simulink model "ur5_simulink_ros2_pbvs_aic"  (R2023b)
settings: Solver=ode4  StartTime=0.0  StopTime=inf  FixedStep=0.005  RelTol=1e-3
model workspace (MAT data in the model file):
  SL_ROS_VariableLengthArrays_MaxSizes.CommonInfo.ArrayTruncateAction = 'EmitWarning'
  SL_ROS_VariableLengthArrays_MaxSizes.MsgTypeMap = containers.Map
  SL_ROS_VariableLengthArrays_MaxSizes.MsgTypeMap.serialization.keys = {'example_interfaces/Float64MultiArray'}
  SL_ROS_VariableLengthArrays_MaxSizes.MsgTypeMap.serialization.values{1}.PropertyName = 'data'
  SL_ROS_VariableLengthArrays_MaxSizes.MsgTypeMap.serialization.values{1}.DataType = 'double'
  SL_ROS_VariableLengthArrays_MaxSizes.MsgTypeMap.serialization.values{1}.MaxLength = 1
  SL_ROS_VariableLengthArrays_MaxSizes.MsgTypeMap.serialization.uniformity = 0
  SL_ROS_VariableLengthArrays_MaxSizes.MsgTypeMap.serialization.keyType = 'char'
  SL_ROS_VariableLengthArrays_MaxSizes.MsgTypeMap.serialization.valueType = 'any'
values from neighbouring files (symbols this model uses):
  D = zeros(6,12)    [ibvs_cstate.m]
undefined symbols (not defined in the file or in its folder): data, data_SL_Info
libraries: ros2lib x8, simulink x3, robotmaniplib x3, robotcorelib x2
settings Model: SimulationMode=accelerator  Creator=81232  LastModifiedBy=ias-lab-701
settings OptimizationCC: EnhancedBackFolding=on  PassReuseOutputArgsAs=Individual arguments  ZeroExternalMemoryAtStartup=off  ZeroInternalMemoryAtStartup=off  MaxStackSize=64  OptimizeBlockOrder=speed  DifferentSizesBufferReuse=on  OptimizationCustomize=off  EfficientTunableParamExpr=on
settings DebuggingCC: ParameterTunabilityLossMsg=error
settings ModelReferenceCC: EnableRefExpFcnMdlSchedulingChecks=on
settings SFSimCC: MATLABDynamicMemAlloc=off
settings RTWCC: Description=Embedded Coder  SystemTargetFile=ert.tlc  HardwareBoard=Robot Operating System 2 (ROS 2)  TLCOptions="-aInlineSetEventsForThisBaseRateFcn=TLC_FALSE -aSuppressMultiTaskScheduler=TLC_FALSE  -aRateBasedStepFcn=0"  TemplateMakefile=ert_default_tmf  Toolchain=Colcon Tools  TargetLang=C++
settings CodeAppCC: ForceParamTrailComments=on  IgnoreCustomStorageClasses=off  OperatorAnnotations=on  SimulinkDataObjDesc=on  SFDataObjDesc=on  InsertBlockDesc=on
settings ERTTargetCC: CodeInterfacePackaging=C++ class  RootIOFormat=Structure reference

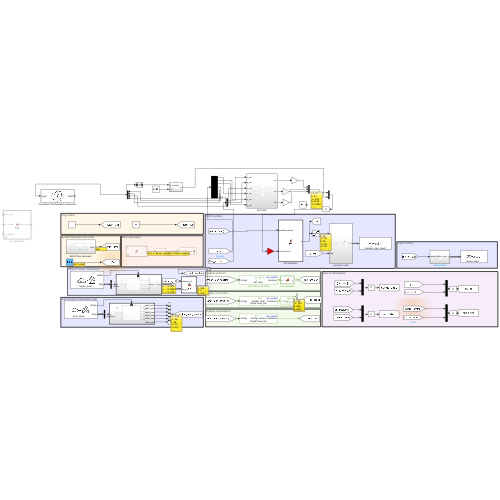
[thumbnail: Simulink's stored preview of the top-level diagram]
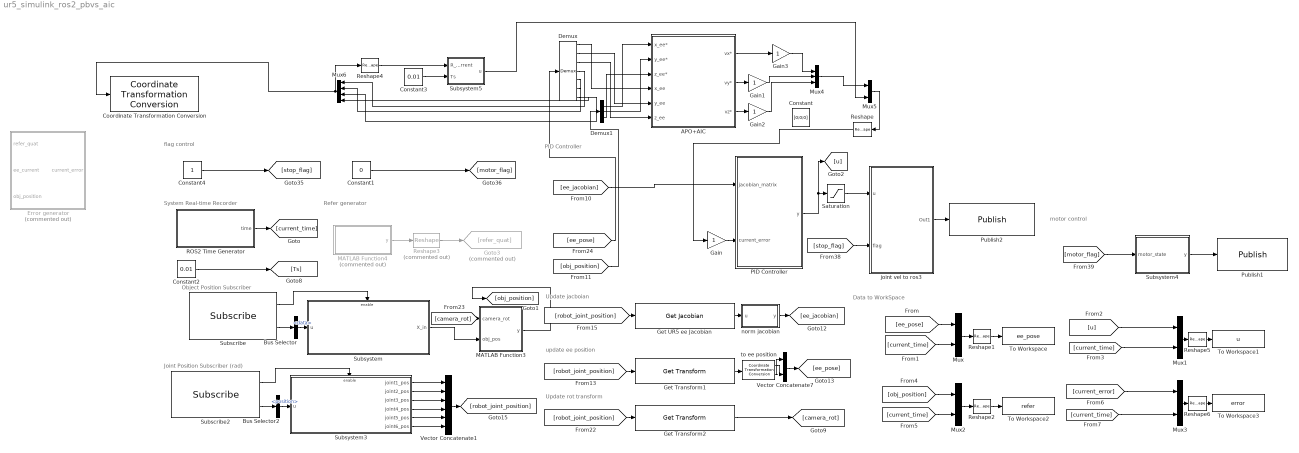
== system ur5_simulink_ros2_pbvs_aic ==
  note: PID Controller
  note: update ee position
  note: Joint Position Subscriber (rad)
  note: Refer generator
  note: Data to WorkSpace
  note: System Real-time Recorder
  note: Object Position Subscriber
  note: Update jacboian
  note: Update rot transform
  note: flag control
  note: motor control
  APO+AIC : Subsystem
  Bus Selector : BusSelector  OutputSignals=data
  Bus Selector2 : BusSelector  OutputSignals=position
  Constant : Constant  Value=[0;0;0]
  Constant1 : Constant  Value=0
  Constant2 : Constant  Value=0.01
  Constant3 : Constant  Value=0.01
  Constant4 : Constant
  Coordinate Transformation Conversion : robotcorelib/Coordinate Transformation Conversion  InputRepresentation=Quaternion  InputEulerSequence=ZYX  ShowTrVecInputPort=on  OutputRepresentation=Rotation Matrix  OutputEulerSequence=ZYX  ShowTrVecOutputPort=on  SimulateUsing=Interpreted execution
  Demux : Demux  Outputs=7
  Demux1 : Demux  Outputs=3
  Error generator : MATLAB Function  Commented=on  TreatAsAtomicUnit=on
  Gain{,1..3} (4 alike) : Gain
  Get Transform1 : robotmaniplib/Get Transform  RigidBodyTree=ur5_model  SourceBody=tool0  TargetBody=base_link  SimulateUsing=Interpreted execution
  Get Transform2 : robotmaniplib/Get Transform  RigidBodyTree=ur5_model  SourceBody=camera  TargetBody=base_link  SimulateUsing=Interpreted execution
  Get UR5 ee Jacobian : robotmaniplib/Get Jacobian  RigidBodyTree=ur5_model  EndEffector=tool0  SimulateUsing=Interpreted execution
  Goto3 : Goto  Commented=on  GotoTag=refer_quat
  MATLAB Function3 : MATLAB Function  TreatAsAtomicUnit=on
  MATLAB Function4 : MATLAB Function  Commented=on  TreatAsAtomicUnit=on
  Mux{,1..3,5} (5 alike) : Mux  Inputs=2
  Mux4 : Mux  Inputs=3
  Mux6 : Mux
  PID Controller : MATLAB Function  TreatAsAtomicUnit=on
  Publish1 : ros2lib/Publish  topicSource=Select from ROS network  topic=/motor_state  messageType=std_msgs/Int64  QOSHistory=Keep last  QOSDepth=1  QOSReliability=Reliable  QOSDurability=Volatile
      settings: LibrarySourceBlock=roslib/ROS 2/Publish
  Publish2 : ros2lib/Publish  topicSource=Select from ROS network  topic=/simulink_mpc_result  messageType=std_msgs/Float64MultiArray  QOSHistory=Keep last  QOSDepth=1  QOSReliability=Reliable  QOSDurability=Volatile
      settings: LibrarySourceBlock=roslib/ROS 2/Publish
  ROS2 Time Generator : Subsystem
  Reshape : Reshape  OutputDimensionality=Customize  OutputDimensions=[6,1]
  Reshape1 : Reshape  OutputDimensionality=Customize  OutputDimensions=[8]
  Reshape2 : Reshape  OutputDimensionality=Customize  OutputDimensions=[4]
  Reshape3 : Reshape  Commented=on  OutputDimensions=[1,7]
  Reshape4 : Reshape  OutputDimensionality=Row vector (2-D)
  Reshape5 : Reshape  OutputDimensionality=Customize  OutputDimensions=[7]
  Reshape6 : Reshape  OutputDimensionality=Customize  OutputDimensions=[7]
  Saturation : Saturate  UpperLimit=0.05  LowerLimit=-0.05  LinearizeAsGain=off
  Subscribe : ros2lib/Subscribe  topicSource=Select from ROS network  topic=/object_pose  messageType=std_msgs/Float64MultiArray  sampleTime=-1  QOSHistory=Keep last  QOSDepth=1  QOSReliability=Reliable  QOSDurability=Volatile
  Subscribe2 : ros2lib/Subscribe  topicSource=Select from ROS network  topic=/joint_states  messageType=sensor_msgs/JointState  sampleTime=-1  QOSHistory=Keep last  QOSDepth=1  QOSReliability=Reliable  QOSDurability=Volatile
  Subsystem : Subsystem
  Subsystem3 : Subsystem
  Subsystem4 : Subsystem
  Subsystem5 : Subsystem
  To Workspace : ToWorkspace  VariableName=ee_pose  SaveFormat=Timeseries  SampleTime=-1
  To Workspace1 : ToWorkspace  VariableName=u  SaveFormat=Timeseries  SampleTime=-1
  To Workspace2 : ToWorkspace  VariableName=refer  SaveFormat=Timeseries  SampleTime=-1
  To Workspace3 : ToWorkspace  VariableName=error  SaveFormat=Timeseries  SampleTime=-1
  Vector Concatenate1 : Concatenate  NumInputs=6
  Vector Concatenate7 : Concatenate
  joint vel to ros3 : Subsystem
  norm jacobian : MATLAB Function  TreatAsAtomicUnit=on
  to ee position : robotcorelib/Coordinate Transformation Conversion  InputRepresentation=Homogeneous Transformation  InputEulerSequence=ZYX  ShowTrVecInputPort=on  OutputRepresentation=Quaternion  OutputEulerSequence=ZYX  ShowTrVecOutputPort=on  SimulateUsing=Interpreted execution
  wires:
  Bus Selector/1 -> Subsystem/1(u)  "<data>"
  Subscribe/2 -> Bus Selector/1
  Subscribe/1 -> Subsystem/Enable
  ROS2 Time Generator/1(time) -> [current_time]
  [ee_pose] -> Mux/1
  [current_time] -> Mux/2
  [current_time] -> Mux1/2
  [current_time] -> Mux2/2
  Mux2/1 -> Reshape2/1
  [current_time] -> Mux3/2
  Mux3/1 -> Reshape6/1
  [current_error] -> Mux3/1
  [u] -> Mux1/1
  Mux1/1 -> Reshape5/1
  Reshape5/1 -> To Workspace1/1
  Reshape6/1 -> To Workspace3/1
  Subscribe2/2 -> Bus Selector2/1
  Bus Selector2/1 -> Subsystem3/1(u)  "<position>"
  Subscribe2/1 -> Subsystem3/Enable
  Subsystem3/1(joint1_pos) -> Vector Concatenate1/1
  Subsystem3/2(joint2_pos) -> Vector Concatenate1/2
  Subsystem3/3(joint3_pos) -> Vector Concatenate1/3
  Subsystem3/4(joint4_pos) -> Vector Concatenate1/4
  Subsystem3/5(joint5_pos) -> Vector Concatenate1/5
  Subsystem3/6(joint6_pos) -> Vector Concatenate1/6
  norm jacobian/1(y) -> [ee_jacobian]
  Get UR5 ee Jacobian/1 -> norm jacobian/1(u)
  [robot_joint_position] -> Get UR5 ee Jacobian/1
  [robot_joint_position] -> Get Transform1/1
  Vector Concatenate1/1 -> [robot_joint_position]
  Mux/1 -> Reshape1/1
  Reshape1/1 -> To Workspace/1
  Reshape2/1 -> To Workspace2/1
  [obj_position] -> Mux2/1
  Constant2/1 -> [Ts]
  Get Transform2/1 -> [camera_rot]
  MATLAB Function3/1(y) -> [obj_position]
  [camera_rot] -> MATLAB Function3/1(camera_rot)
  Subsystem/1(X_in) -> MATLAB Function3/2(obj_pos)
  Reshape3/1 -> Goto3/1
  MATLAB Function4/1(y) -> Reshape3/1
  Get Transform1/1 -> to ee position/1
  to ee position/1 -> Vector Concatenate7/2
  to ee position/2 -> Vector Concatenate7/1
  Vector Concatenate7/1 -> [ee_pose]
  [ee_jacobian] -> PID Controller/1(jacobian_matrix)
  Saturation/1 -> joint vel to ros3/1(u)
  joint vel to ros3/1(Out1) -> Publish2/1
  PID Controller/1(y) -> Saturation/1, [u]
  Constant4/1 -> [stop_flag]
  [stop_flag] -> joint vel to ros3/2(flag)
  Mux5/1 -> Reshape/1
  Gain/1 -> PID Controller/2(current_error)
  Subsystem4/1(y) -> Publish1/1
  [motor_flag] -> Subsystem4/1(motor_state)
  Constant1/1 -> [motor_flag]
  [robot_joint_position] -> Get Transform2/1
  Demux/1 -> APO+AIC/4(x_ee)
  Demux/2 -> APO+AIC/5(y_ee)
  Demux/3 -> APO+AIC/6(z_ee)
  Demux1/1 -> APO+AIC/1(x_ee*)
  Demux1/2 -> APO+AIC/2(y_ee*)
  Demux1/3 -> APO+AIC/3(z_ee*)
  APO+AIC/1(vx*) -> Gain3/1
  APO+AIC/3(vz*) -> Gain2/1
  Mux4/1 -> Mux5/1
  Reshape/1 -> Gain/1
  [ee_pose] -> Demux/1
  [obj_position] -> Demux1/1
  APO+AIC/2(vy*) -> Gain1/1
  Gain1/1 -> Mux4/2
  Gain2/1 -> Mux4/3
  Gain3/1 -> Mux4/1
  Constant3/1 -> Subsystem5/2(Ts)
  Demux/4 -> Mux6/1
  Demux/5 -> Mux6/2
  Demux/6 -> Mux6/3
  Demux/7 -> Mux6/4
  Mux6/1 -> Reshape4/1, Coordinate Transformation Conversion/1
  Subsystem5/1(u) -> Mux5/2
  Reshape4/1 -> Subsystem5/1(R_current)

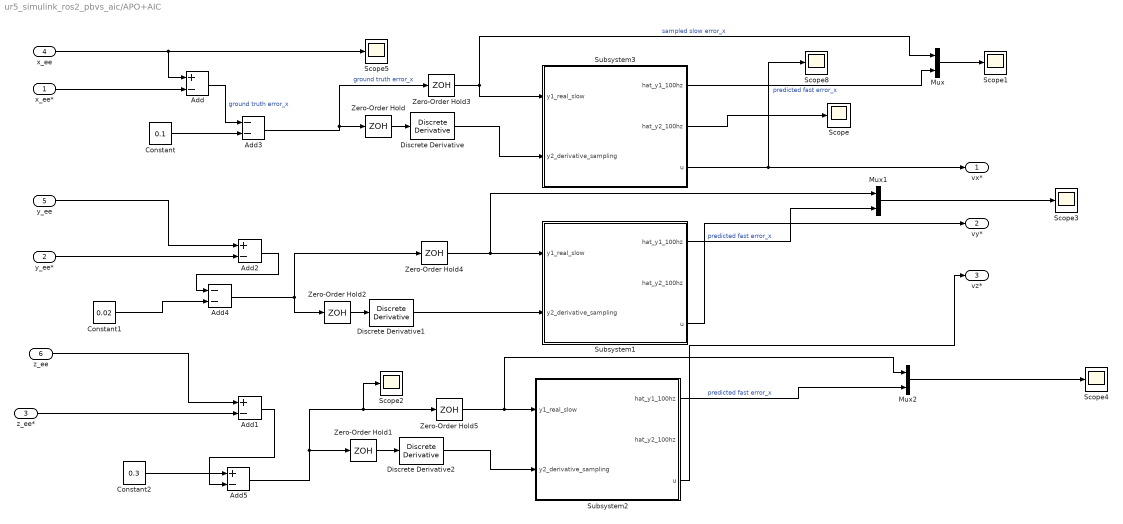
== system ur5_simulink_ros2_pbvs_aic/APO+AIC ==
  x_ee* : Inport
  y_ee* : Inport  Port=2
  z_ee* : Inport  Port=3
  x_ee : Inport  Port=4
  y_ee : Inport  Port=5
  z_ee : Inport  Port=6
  Add{,1..2,5} (4 alike) : Sum  Inputs=+-
  Add3 : Sum  Inputs=--
  Add4 : Sum  Inputs=--
  Constant : Constant  Value=0.1
  Constant1 : Constant  Value=0.02
  Constant2 : Constant  Value=0.3
  Discrete Derivative : simulink/Discrete/Discrete Derivative  gainval=1.0  ICPrevScaledInput=0  OutMin=[]  OutMax=[]  OutDataType=fixdt(1, 16)  OutScaling=2^-10  DoSatur=off
  Discrete Derivative1 : simulink/Discrete/Discrete Derivative  gainval=1.0  ICPrevScaledInput=0.0  OutMin=[]  OutMax=[]  OutDataType=fixdt(1, 16)  OutScaling=2^-10  DoSatur=off
  Discrete Derivative2 : simulink/Discrete/Discrete Derivative  gainval=1.0  ICPrevScaledInput=0.0  OutMin=[]  OutMax=[]  OutDataType=fixdt(1, 16)  OutScaling=2^-10  DoSatur=off
  Mux : Mux  Inputs=2
  Mux1 : Mux  Inputs=2
  Mux2 : Mux  Inputs=2
  Scope{,1..5,8} (7 alike) : Scope
  Subsystem1 : Subsystem
  Subsystem2 : Subsystem
  Subsystem3 : Subsystem
  Zero-Order Hold{,1..5} (6 alike) : ZeroOrderHold  SampleTime=0.05
  vx* : Outport
  vy* : Outport  Port=2
  vz* : Outport  Port=3
  wires:
  Add4/1 -> Zero-Order Hold4/1, Zero-Order Hold2/1
  x_ee/1 -> Scope5/1, Add/1
  Discrete Derivative/1 -> Subsystem3/2(y2_derivative_sampling)
  Zero-Order Hold/1 -> Discrete Derivative/1
  Discrete Derivative1/1 -> Subsystem1/2(y2_derivative_sampling)
  Add5/1 -> Zero-Order Hold5/1, Scope2/1, Zero-Order Hold1/1
  Subsystem3/3(u) -> vx*/1, Scope8/1
  Add3/1 -> Zero-Order Hold3/1, Zero-Order Hold/1  "ground truth error_x"
  x_ee*/1 -> Add/2
  y_ee/1 -> Add2/1
  z_ee/1 -> Add1/1
  Subsystem2/3(u) -> vz*/1
  Zero-Order Hold1/1 -> Discrete Derivative2/1
  Zero-Order Hold2/1 -> Discrete Derivative1/1
  y_ee*/1 -> Add2/2
  z_ee*/1 -> Add1/2
  Zero-Order Hold3/1 -> Mux/1, Subsystem3/1(y1_real_slow)  "sampled slow error_x"
  Zero-Order Hold4/1 -> Mux1/1, Subsystem1/1(y1_real_slow)
  Subsystem1/3(u) -> vy*/1
  Subsystem3/1(hat_y1_100hz) -> Mux/2  "predicted fast error_x"
  Mux/1 -> Scope1/1
  Discrete Derivative2/1 -> Subsystem2/2(y2_derivative_sampling)
  Add/1 -> Add3/1  "ground truth error_x"
  Constant/1 -> Add3/2
  Constant1/1 -> Add4/2
  Add2/1 -> Add4/1
  Constant2/1 -> Add5/1
  Add1/1 -> Add5/2
  Subsystem3/2(hat_y2_100hz) -> Scope/1
  Subsystem1/1(hat_y1_100hz) -> Mux1/2  "predicted fast error_x"
  Mux1/1 -> Scope3/1
  Mux2/1 -> Scope4/1
  Zero-Order Hold5/1 -> Mux2/1, Subsystem2/1(y1_real_slow)
  Subsystem2/1(hat_y1_100hz) -> Mux2/2  "predicted fast error_x"

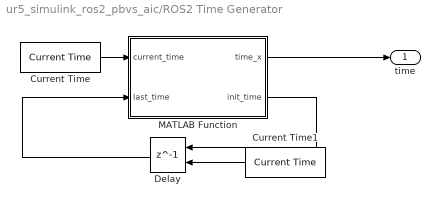
== system ur5_simulink_ros2_pbvs_aic/ROS2 Time Generator ==
  Current Time : ros2lib/Current Time  OutputFormat=double  SampleTime=-1  ModelName=ur5_simulink_ros2_pbvs_aic
      settings: LibrarySourceBlock=roslib/ROS 2/Current Time
  Current Time1 : ros2lib/Current Time  OutputFormat=double  SampleTime=-1  ModelName=ur5_simulink_ros2_pbvs_aic
      settings: LibrarySourceBlock=roslib/ROS 2/Current Time
  Delay : Delay  DelayLength=1  InitialConditionSource=Input port
      settings: InputPortMap=u0,p4
  MATLAB Function : MATLAB Function  TreatAsAtomicUnit=on
  time : Outport
  wires:
  Delay/1 -> MATLAB Function/2(last_time)
  Current Time1/1 -> Delay/2
  MATLAB Function/2(init_time) -> Delay/1
  Current Time/1 -> MATLAB Function/1(current_time)
  MATLAB Function/1(time_x) -> time/1

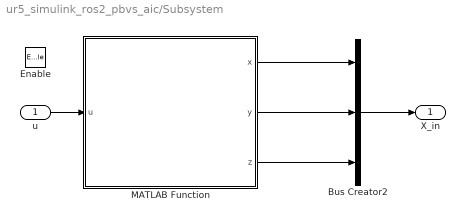
== system ur5_simulink_ros2_pbvs_aic/Subsystem ==
  u : Inport
  Enable : EnablePort
  Bus Creator2 : BusCreator  Inputs=3
  MATLAB Function : MATLAB Function  TreatAsAtomicUnit=on
  X_in : Outport
  wires:
  MATLAB Function/2(y) -> Bus Creator2/2
  MATLAB Function/1(x) -> Bus Creator2/1
  MATLAB Function/3(z) -> Bus Creator2/3
  u/1 -> MATLAB Function/1(u)
  Bus Creator2/1 -> X_in/1

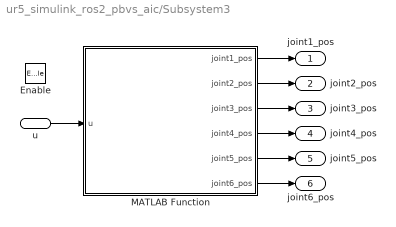
== system ur5_simulink_ros2_pbvs_aic/Subsystem3 ==
  u : Inport
  Enable : EnablePort
  MATLAB Function : MATLAB Function  TreatAsAtomicUnit=on
  joint1_pos : Outport
  joint2_pos : Outport  Port=2
  joint3_pos : Outport  Port=3
  joint4_pos : Outport  Port=4
  joint5_pos : Outport  Port=5
  joint6_pos : Outport  Port=6
  wires:
  u/1 -> MATLAB Function/1(u)
  MATLAB Function/1(joint1_pos) -> joint1_pos/1
  MATLAB Function/2(joint2_pos) -> joint2_pos/1
  MATLAB Function/3(joint3_pos) -> joint3_pos/1
  MATLAB Function/4(joint4_pos) -> joint4_pos/1
  MATLAB Function/5(joint5_pos) -> joint5_pos/1
  MATLAB Function/6(joint6_pos) -> joint6_pos/1

== system ur5_simulink_ros2_pbvs_aic/Subsystem4 ==
  motor_state : Inport
  Blank Message : ros2lib/Blank Message  messageClass=Message  entityType=std_msgs/Int64  messageType=std_msgs/Int64  SampleTime=inf
  Bus Assignment1 : BusAssignment  AssignedSignals=data
  y : Outport
  wires:
  Blank Message/1 -> Bus Assignment1/1
  Bus Assignment1/1 -> y/1
  motor_state/1 -> Bus Assignment1/2

== system ur5_simulink_ros2_pbvs_aic/Subsystem5 ==
  R_current : Inport
  Ts : Inport  Port=2
  Discrete Pulse Generator : DiscretePulseGenerator  SampleTime=0.005
  attitude_pi_ctrl : Subsystem
  u : Outport
  wires:
  Ts/1 -> attitude_pi_ctrl/2(Ts)
  Discrete Pulse Generator/1 -> attitude_pi_ctrl/Trigger
  R_current/1 -> attitude_pi_ctrl/1(R_current)
  attitude_pi_ctrl/1(u) -> u/1

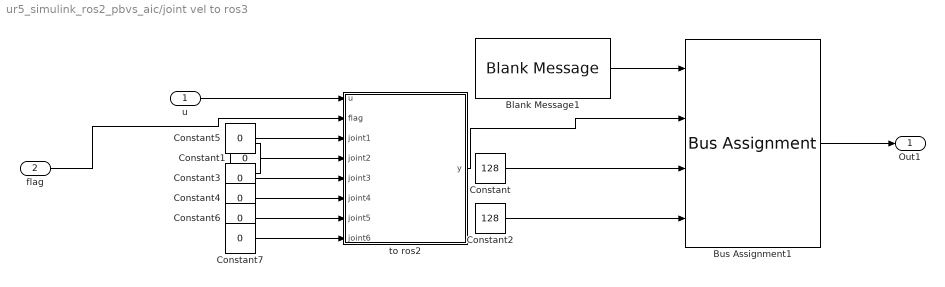
== system ur5_simulink_ros2_pbvs_aic/joint vel to ros3 ==
  u : Inport
  flag : Inport  Port=2
  Blank Message1 : ros2lib/Blank Message  messageClass=Message  entityType=std_msgs/Float64MultiArray  messageType=std_msgs/Float64MultiArray  SampleTime=inf
      settings: LibrarySourceBlock=roslib/ROS 2/Blank Message
  Bus Assignment1 : BusAssignment  AssignedSignals=data,data_SL_Info.CurrentLength,data_SL_Info.ReceivedLength
  Constant : Constant  Value=128  OutDataTypeStr=uint32
  Constant{1,3..7} (6 alike) : Constant  Value=0
  Constant2 : Constant  Value=128  OutDataTypeStr=uint32
  to ros2 : MATLAB Function  TreatAsAtomicUnit=on
  Out1 : Outport
  wires:
  u/1 -> to ros2/1(u)
  Constant2/1 -> Bus Assignment1/4
  Constant/1 -> Bus Assignment1/3
  Blank Message1/1 -> Bus Assignment1/1
  Bus Assignment1/1 -> Out1/1
  Constant5/1 -> to ros2/3(joint1)
  Constant1/1 -> to ros2/4(joint2)
  Constant3/1 -> to ros2/5(joint3)
  Constant4/1 -> to ros2/6(joint4)
  Constant6/1 -> to ros2/7(joint5)
  Constant7/1 -> to ros2/8(joint6)
  flag/1 -> to ros2/2(flag)
  to ros2/1(y) -> Bus Assignment1/2

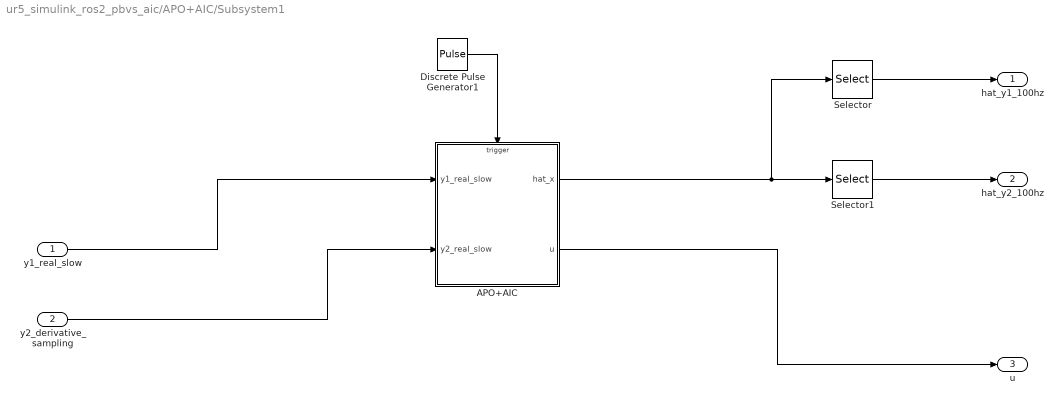
== system ur5_simulink_ros2_pbvs_aic/APO+AIC/Subsystem1 ==
  y1_real_slow : Inport
  y2_derivative_sampling : Inport  Port=2
  APO+AIC : Subsystem
  Discrete Pulse Generator1 : DiscretePulseGenerator  SampleTime=0.005
  Selector : Selector  InputPortWidth=2  IndexOptions=Index vector (dialog)  Indices=[1]  OutputSizes=1
  Selector1 : Selector  InputPortWidth=2  IndexOptions=Index vector (dialog)  Indices=[2]  OutputSizes=1
  hat_y1_100hz : Outport
  hat_y2_100hz : Outport  Port=2
  u : Outport  Port=3
  wires:
  y1_real_slow/1 -> APO+AIC/1(y1_real_slow)
  y2_derivative_sampling/1 -> APO+AIC/2(y2_real_slow)
  Selector1/1 -> hat_y2_100hz/1
  Discrete Pulse Generator1/1 -> APO+AIC/Trigger
  APO+AIC/1(hat_x) -> Selector/1, Selector1/1
  Selector/1 -> hat_y1_100hz/1
  APO+AIC/2(u) -> u/1

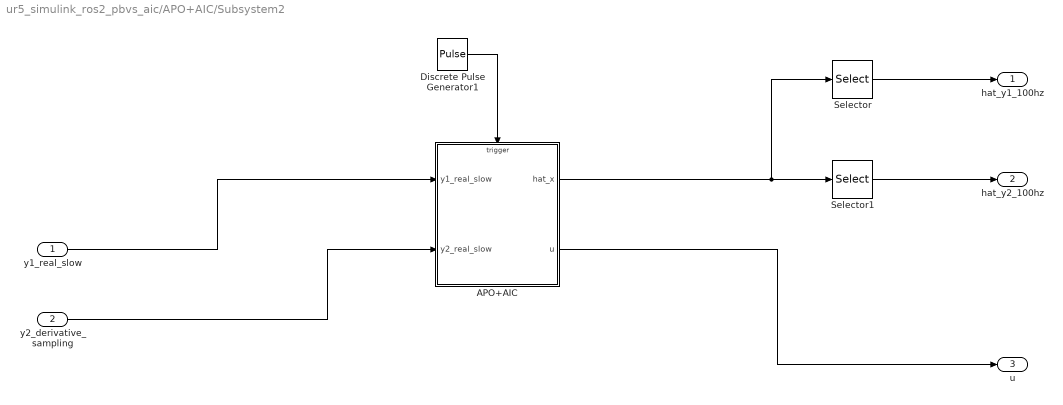
== system ur5_simulink_ros2_pbvs_aic/APO+AIC/Subsystem2 ==
  y1_real_slow : Inport
  y2_derivative_sampling : Inport  Port=2
  APO+AIC : Subsystem
  Discrete Pulse Generator1 : DiscretePulseGenerator  SampleTime=0.005
  Selector : Selector  InputPortWidth=2  IndexOptions=Index vector (dialog)  Indices=[1]  OutputSizes=1
  Selector1 : Selector  InputPortWidth=2  IndexOptions=Index vector (dialog)  Indices=[2]  OutputSizes=1
  hat_y1_100hz : Outport
  hat_y2_100hz : Outport  Port=2
  u : Outport  Port=3
  wires:
  y1_real_slow/1 -> APO+AIC/1(y1_real_slow)
  y2_derivative_sampling/1 -> APO+AIC/2(y2_real_slow)
  Selector1/1 -> hat_y2_100hz/1
  Discrete Pulse Generator1/1 -> APO+AIC/Trigger
  APO+AIC/1(hat_x) -> Selector/1, Selector1/1
  Selector/1 -> hat_y1_100hz/1
  APO+AIC/2(u) -> u/1

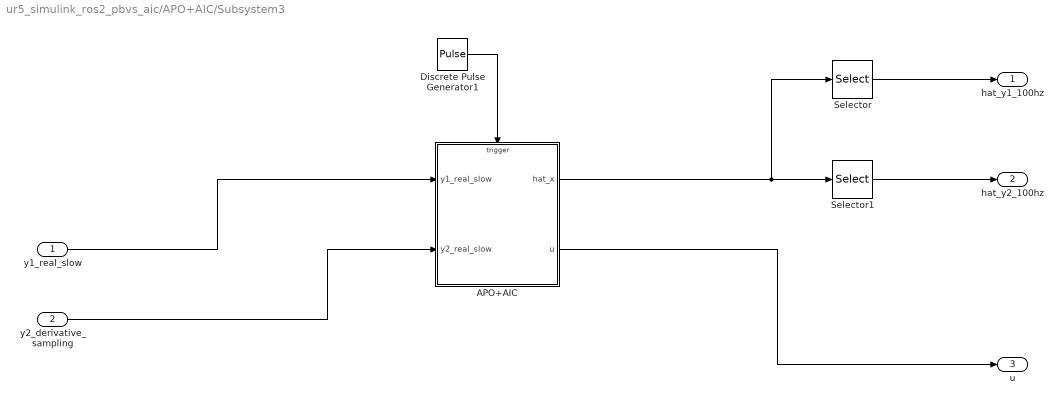
== system ur5_simulink_ros2_pbvs_aic/APO+AIC/Subsystem3 ==
  y1_real_slow : Inport
  y2_derivative_sampling : Inport  Port=2
  APO+AIC : Subsystem
  Discrete Pulse Generator1 : DiscretePulseGenerator  SampleTime=0.005
  Selector : Selector  InputPortWidth=2  IndexOptions=Index vector (dialog)  Indices=[1]  OutputSizes=1
  Selector1 : Selector  InputPortWidth=2  IndexOptions=Index vector (dialog)  Indices=[2]  OutputSizes=1
  hat_y1_100hz : Outport
  hat_y2_100hz : Outport  Port=2
  u : Outport  Port=3
  wires:
  y1_real_slow/1 -> APO+AIC/1(y1_real_slow)
  y2_derivative_sampling/1 -> APO+AIC/2(y2_real_slow)
  Selector1/1 -> hat_y2_100hz/1
  Discrete Pulse Generator1/1 -> APO+AIC/Trigger
  APO+AIC/1(hat_x) -> Selector/1, Selector1/1
  Selector/1 -> hat_y1_100hz/1
  APO+AIC/2(u) -> u/1

== system ur5_simulink_ros2_pbvs_aic/Subsystem5/attitude_pi_ctrl ==
  R_current : Inport
  Ts : Inport  Port=2
  Trigger : TriggerPort  VariantControl=(inherit)  PortDimensions=1
  Subsystem : Subsystem
  u : Outport
  wires:
  R_current/1 -> Subsystem/1(R_current)
  Ts/1 -> Subsystem/2(Ts)
  Subsystem/1(u) -> u/1

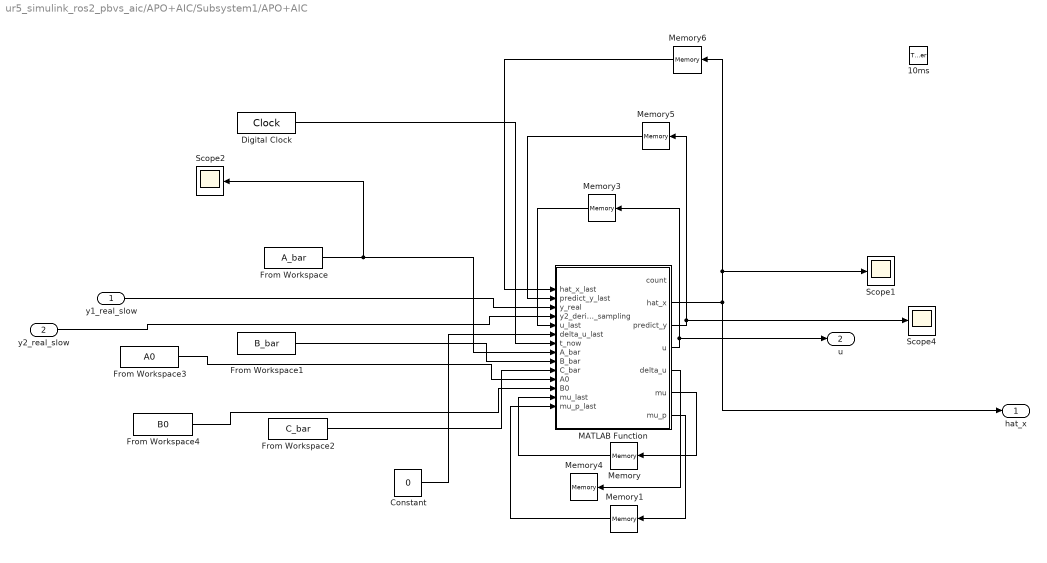
== system ur5_simulink_ros2_pbvs_aic/APO+AIC/Subsystem1/APO+AIC ==
  y1_real_slow : Inport
  y2_real_slow : Inport  Port=2
  10ms : TriggerPort  VariantControl=(inherit)  InitialTriggerSignalState=zero  PortDimensions=1
  Constant : Constant  Value=0
  Digital Clock : DigitalClock  SampleTime=-1
  From Workspace : FromWorkspace  VariableName=A_bar  OutDataTypeStr=double  SampleTime=-1  OutputAfterFinalValue=Holding final value
  From Workspace1 : FromWorkspace  VariableName=B_bar  OutDataTypeStr=double  SampleTime=-1  OutputAfterFinalValue=Holding final value
  From Workspace2 : FromWorkspace  VariableName=C_bar  OutDataTypeStr=double  SampleTime=-1  OutputAfterFinalValue=Holding final value
  From Workspace3 : FromWorkspace  VariableName=A0  OutDataTypeStr=double  SampleTime=-1  OutputAfterFinalValue=Holding final value
  From Workspace4 : FromWorkspace  VariableName=B0  OutDataTypeStr=double  SampleTime=-1  OutputAfterFinalValue=Holding final value
  MATLAB Function : MATLAB Function  TreatAsAtomicUnit=on
  Memory{,1,3..6} (6 alike) : Memory  InheritSampleTime=on
  Scope1 : Scope
  Scope2 : Scope
  Scope4 : Scope
  hat_x : Outport
  u : Outport  Port=2
  wires:
  From Workspace2/1 -> MATLAB Function/10(C_bar)
  From Workspace1/1 -> MATLAB Function/9(B_bar)
  Digital Clock/1 -> MATLAB Function/7(t_now)
  Memory5/1 -> MATLAB Function/2(predict_y_last)
  MATLAB Function/3(predict_y) -> Memory5/1, Scope4/1
  From Workspace/1 -> Scope2/1, MATLAB Function/8(A_bar)
  MATLAB Function/2(hat_x) -> Memory6/1, Scope1/1, hat_x/1
  y1_real_slow/1 -> MATLAB Function/3(y_real)
  From Workspace3/1 -> MATLAB Function/11(A0)
  From Workspace4/1 -> MATLAB Function/12(B0)
  MATLAB Function/6(mu) -> Memory/1
  Memory/1 -> MATLAB Function/13(mu_last)
  MATLAB Function/7(mu_p) -> Memory1/1
  Memory1/1 -> MATLAB Function/14(mu_p_last)
  y2_real_slow/1 -> MATLAB Function/4(y2_derivative_sampling)
  MATLAB Function/4(u) -> Memory3/1, u/1
  Memory3/1 -> MATLAB Function/5(u_last)
  MATLAB Function/5(delta_u) -> Memory4/1
  Memory6/1 -> MATLAB Function/1(hat_x_last)
  Constant/1 -> MATLAB Function/6(delta_u_last)

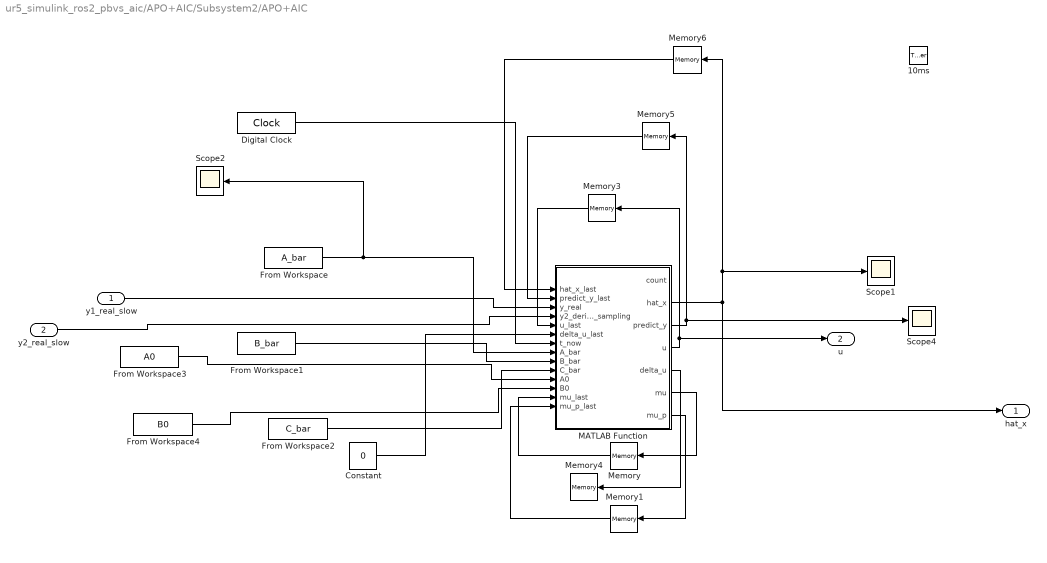
== system ur5_simulink_ros2_pbvs_aic/APO+AIC/Subsystem2/APO+AIC ==
  y1_real_slow : Inport
  y2_real_slow : Inport  Port=2
  10ms : TriggerPort  VariantControl=(inherit)  InitialTriggerSignalState=zero  PortDimensions=1
  Constant : Constant  Value=0
  Digital Clock : DigitalClock  SampleTime=-1
  From Workspace : FromWorkspace  VariableName=A_bar  OutDataTypeStr=double  SampleTime=-1  OutputAfterFinalValue=Holding final value
  From Workspace1 : FromWorkspace  VariableName=B_bar  OutDataTypeStr=double  SampleTime=-1  OutputAfterFinalValue=Holding final value
  From Workspace2 : FromWorkspace  VariableName=C_bar  OutDataTypeStr=double  SampleTime=-1  OutputAfterFinalValue=Holding final value
  From Workspace3 : FromWorkspace  VariableName=A0  OutDataTypeStr=double  SampleTime=-1  OutputAfterFinalValue=Holding final value
  From Workspace4 : FromWorkspace  VariableName=B0  OutDataTypeStr=double  SampleTime=-1  OutputAfterFinalValue=Holding final value
  MATLAB Function : MATLAB Function  TreatAsAtomicUnit=on
  Memory{,1,3..6} (6 alike) : Memory  InheritSampleTime=on
  Scope1 : Scope
  Scope2 : Scope
  Scope4 : Scope
  hat_x : Outport
  u : Outport  Port=2
  wires:
  From Workspace2/1 -> MATLAB Function/10(C_bar)
  From Workspace1/1 -> MATLAB Function/9(B_bar)
  Digital Clock/1 -> MATLAB Function/7(t_now)
  Memory5/1 -> MATLAB Function/2(predict_y_last)
  MATLAB Function/3(predict_y) -> Memory5/1, Scope4/1
  From Workspace/1 -> Scope2/1, MATLAB Function/8(A_bar)
  MATLAB Function/2(hat_x) -> Memory6/1, Scope1/1, hat_x/1
  y1_real_slow/1 -> MATLAB Function/3(y_real)
  From Workspace3/1 -> MATLAB Function/11(A0)
  From Workspace4/1 -> MATLAB Function/12(B0)
  MATLAB Function/6(mu) -> Memory/1
  Memory/1 -> MATLAB Function/13(mu_last)
  MATLAB Function/7(mu_p) -> Memory1/1
  Memory1/1 -> MATLAB Function/14(mu_p_last)
  y2_real_slow/1 -> MATLAB Function/4(y2_derivative_sampling)
  MATLAB Function/4(u) -> Memory3/1, u/1
  Memory3/1 -> MATLAB Function/5(u_last)
  MATLAB Function/5(delta_u) -> Memory4/1
  Memory6/1 -> MATLAB Function/1(hat_x_last)
  Constant/1 -> MATLAB Function/6(delta_u_last)

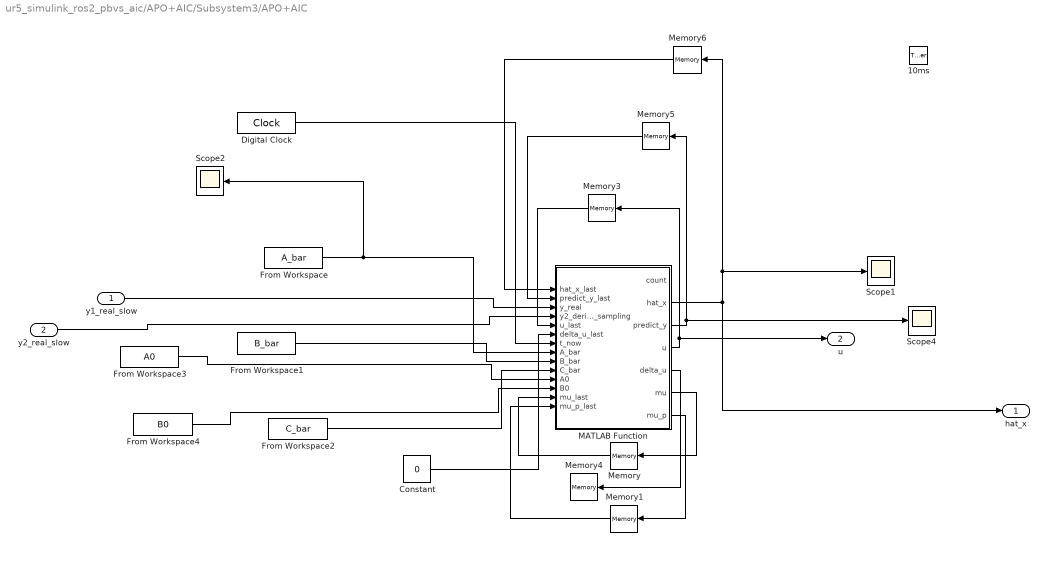
== system ur5_simulink_ros2_pbvs_aic/APO+AIC/Subsystem3/APO+AIC ==
  y1_real_slow : Inport
  y2_real_slow : Inport  Port=2
  10ms : TriggerPort  VariantControl=(inherit)  InitialTriggerSignalState=zero  PortDimensions=1
  Constant : Constant  Value=0
  Digital Clock : DigitalClock  SampleTime=-1
  From Workspace : FromWorkspace  VariableName=A_bar  OutDataTypeStr=double  SampleTime=-1  OutputAfterFinalValue=Holding final value
  From Workspace1 : FromWorkspace  VariableName=B_bar  OutDataTypeStr=double  SampleTime=-1  OutputAfterFinalValue=Holding final value
  From Workspace2 : FromWorkspace  VariableName=C_bar  OutDataTypeStr=double  SampleTime=-1  OutputAfterFinalValue=Holding final value
  From Workspace3 : FromWorkspace  VariableName=A0  OutDataTypeStr=double  SampleTime=-1  OutputAfterFinalValue=Holding final value
  From Workspace4 : FromWorkspace  VariableName=B0  OutDataTypeStr=double  SampleTime=-1  OutputAfterFinalValue=Holding final value
  MATLAB Function : MATLAB Function  TreatAsAtomicUnit=on
  Memory{,1,3..6} (6 alike) : Memory  InheritSampleTime=on
  Scope1 : Scope
  Scope2 : Scope
  Scope4 : Scope
  hat_x : Outport
  u : Outport  Port=2
  wires:
  From Workspace2/1 -> MATLAB Function/10(C_bar)
  From Workspace1/1 -> MATLAB Function/9(B_bar)
  Digital Clock/1 -> MATLAB Function/7(t_now)
  Memory5/1 -> MATLAB Function/2(predict_y_last)
  MATLAB Function/3(predict_y) -> Memory5/1, Scope4/1
  From Workspace/1 -> Scope2/1, MATLAB Function/8(A_bar)
  MATLAB Function/2(hat_x) -> Memory6/1, Scope1/1, hat_x/1
  y1_real_slow/1 -> MATLAB Function/3(y_real)
  From Workspace3/1 -> MATLAB Function/11(A0)
  From Workspace4/1 -> MATLAB Function/12(B0)
  MATLAB Function/6(mu) -> Memory/1
  Memory/1 -> MATLAB Function/13(mu_last)
  MATLAB Function/7(mu_p) -> Memory1/1
  Memory1/1 -> MATLAB Function/14(mu_p_last)
  y2_real_slow/1 -> MATLAB Function/4(y2_derivative_sampling)
  MATLAB Function/4(u) -> Memory3/1, u/1
  Memory3/1 -> MATLAB Function/5(u_last)
  MATLAB Function/5(delta_u) -> Memory4/1
  Memory6/1 -> MATLAB Function/1(hat_x_last)
  Constant/1 -> MATLAB Function/6(delta_u_last)

== system ur5_simulink_ros2_pbvs_aic/Subsystem5/attitude_pi_ctrl/Subsystem ==
  R_current : Inport
  Ts : Inport  Port=2
  MATLAB Function : MATLAB Function  TreatAsAtomicUnit=on
  u : Outport
  wires:
  Ts/1 -> MATLAB Function/2(Ts)
  MATLAB Function/1(u) -> u/1
  R_current/1 -> MATLAB Function/1(R_current)

== matlab function ur5_simulink_ros2_pbvs_aic/norm jacobian ==
  data: u input; y output size=[6,6]
function y = fcn(u)
firstThreeColumns =u(1:3, :);
lastThreeColumns = u(4:6, :);
y = [lastThreeColumns;firstThreeColumns];

== matlab function ur5_simulink_ros2_pbvs_aic/Subsystem3/MATLAB Function ==
  data: u input; joint1_pos output; joint2_pos output; joint3_pos output; joint4_pos output; joint5_pos output; joint6_pos output
function [joint1_pos,joint2_pos,joint3_pos,joint4_pos,joint5_pos,joint6_pos] = fcn(u)
joint1_pos = u(6);
joint2_pos = u(1);
joint3_pos = u(2);
joint4_pos = u(3);
joint5_pos = u(4);
joint6_pos = u(5);

== matlab function ur5_simulink_ros2_pbvs_aic/APO+AIC/Subsystem2/APO+AIC/MATLAB Function ==
  data: count output; hat_x_last input; predict_y_last input; y_real input; y2_derivative_sampling input; u_last input; delta_u_last input; hat_x output; t_now input; A_bar input; B_bar input; C_bar input; predict_y output; A0 input; B0 input; mu_last input; mu_p_last input; u output; delta_u output; mu output; mu_p output
function [count,hat_x,predict_y, u, delta_u, mu, mu_p] = fcn(hat_x_last, predict_y_last, y_real,y2_derivative_sampling, u_last,delta_u_last,t_now,A_bar,B_bar,C_bar,A0,B0,mu_last, mu_p_last)
if(t_now==0)
    count=0;
    hat_x = zeros(2,1);
    predict_y = y_real;
    hat_x(1,1)=y_real;
    [u, delta_u, mu, mu_p]  = AIC2(t_now, 1, y_real,hat_x(1,1),y2_derivative_sampling,hat_x(2,1), mu_last, mu_p_last, u_last);
else
    count=mod(t_now,0.05);
    if(count==0)%在采样的时刻
        predict_y=y_real;
        hat_x=A_bar*hat_x_last +B_bar*delta_u_last/0.01+ C_bar*predict_y;
        [u, delta_u, mu, mu_p]  = AIC2(t_now, 1, y_real,hat_x(1,1),y2_derivative_sampling,hat_x(2,1), mu_last, mu_p_last, u_last);
    else%在两个采样时刻之间
        predict_y=[1 0]*(A0*hat_x_last+B0*delta_u_last);
        hat_x=A_bar*hat_x_last + B_bar*delta_u_last/0.01+C_bar*predict_y_last;
        [u, delta_u, mu, mu_p]  = AIC2(t_now, 1, y_real,hat_x(1,1),y2_derivative_sampling,hat_x(2,1), mu_last, mu_p_last, u_last);
    end
end
end








% function [count,hat_x,predict_y, u, delta_u, mu, mu_p, mu_pp] = fcn(hat_x_last, predict_y_last, y_real,y2_derivative_sampling,y3_real_slow, u_last,delta_u_last,t_now,A_bar,B_bar,C_bar,A0,B0,mu_last, mu_p_last, mu_pp_last)
% if(t_now==0)
%     count=0;
%     hat_x = zeros(3,1);
%     predict_y = y_real;
%     hat_x(1,1)=y_real;
%     u_now=0;
%     hat_x = A_bar*hat_x + B_bar*u_now+ C_bar*predict_y;
%     [u, delta_u, mu, mu_p, mu_pp]  = AIC3(t_now, 1, y_real,hat_x(1,1),y2_derivative_sampling,hat_x(2,1), y3_real_slow, hat_x(3,1), mu_last, mu_p_last, mu_pp_last, u_last);
%     %predict_y=[1 0 0]*(A0*hat_x+B0*delta_u); 
%     
% else
%     count=mod(t_now,0.05);
%     if(count==0)%在采样的时刻
%         predict_y=y_real;
%         hat_x=A_bar*hat_x_last +B_bar*delta_u_last+ C_bar*predict_y;
%         %hat_x(1,1)=y_real;
%         [u, delta_u, mu, mu_p, mu_pp]  = AIC3(t_now, 1, y_real,hat_x(1,1),y2_derivative_sampling,hat_x(2,1), y3_real_slow, hat_x(3,1), mu_last, mu_p_last, mu_pp_last, u_last);
% 
%         %predict_y=[1 0 0]*(A0*hat_x+B0*delta_u);
%         
%     else%在两个采样时刻之间
%         predict_y=[1 0 0]*(A0*hat_x_last+B0*delta_u_last);
%         hat_x=A_bar*hat_x_last + B_bar*delta_u_last+C_bar*predict_y_last;
%         [u, delta_u, mu, mu_p, mu_pp]  = AIC3(t_now, 1, y_real,hat_x(1,1),y2_derivative_sampling,hat_x(2,1), y3_real_slow, hat_x(3,1), mu_last, mu_p_last, mu_pp_last, u_last);
%         %predict_y=[1 0 0]*(A0*hat_x+B0*delta_u);
%         
%     end
% end
% end

== matlab function ur5_simulink_ros2_pbvs_aic/APO+AIC/Subsystem3/APO+AIC/MATLAB Function ==
  data: count output; hat_x_last input; predict_y_last input; y_real input; y2_derivative_sampling input; u_last input; delta_u_last input; hat_x output; t_now input; A_bar input; B_bar input; C_bar input; predict_y output; A0 input; B0 input; mu_last input; mu_p_last input; u output; delta_u output; mu output; mu_p output
function [count,hat_x,predict_y, u, delta_u, mu, mu_p] = fcn(hat_x_last, predict_y_last, y_real,y2_derivative_sampling, u_last,delta_u_last,t_now,A_bar,B_bar,C_bar,A0,B0,mu_last, mu_p_last)
if(t_now==0)
    count=0;
    hat_x = zeros(2,1);
    predict_y = y_real;
    hat_x(1,1)=y_real;
    [u, delta_u, mu, mu_p]  = AIC2(t_now, 1, y_real,hat_x(1,1),y2_derivative_sampling,hat_x(2,1), mu_last, mu_p_last, u_last);
else
    count=mod(t_now,0.05);
    if(count==0)%在采样的时刻
        predict_y=y_real;
        hat_x=A_bar*hat_x_last +B_bar*delta_u_last/0.01+ C_bar*predict_y;
        [u, delta_u, mu, mu_p]  = AIC2(t_now, 1, y_real,hat_x(1,1),y2_derivative_sampling,hat_x(2,1), mu_last, mu_p_last, u_last);
    else%在两个采样时刻之间
        predict_y=[1 0]*(A0*hat_x_last+B0*delta_u_last);
        hat_x=A_bar*hat_x_last + B_bar*delta_u_last/0.01+C_bar*predict_y_last;
        [u, delta_u, mu, mu_p]  = AIC2(t_now, 1, y_real,hat_x(1,1),y2_derivative_sampling,hat_x(2,1), mu_last, mu_p_last, u_last);
    end
end
end








% function [count,hat_x,predict_y, u, delta_u, mu, mu_p, mu_pp] = fcn(hat_x_last, predict_y_last, y_real,y2_derivative_sampling,y3_real_slow, u_last,delta_u_last,t_now,A_bar,B_bar,C_bar,A0,B0,mu_last, mu_p_last, mu_pp_last)
% if(t_now==0)
%     count=0;
%     hat_x = zeros(3,1);
%     predict_y = y_real;
%     hat_x(1,1)=y_real;
%     u_now=0;
%     hat_x = A_bar*hat_x + B_bar*u_now+ C_bar*predict_y;
%     [u, delta_u, mu, mu_p, mu_pp]  = AIC3(t_now, 1, y_real,hat_x(1,1),y2_derivative_sampling,hat_x(2,1), y3_real_slow, hat_x(3,1), mu_last, mu_p_last, mu_pp_last, u_last);
%     %predict_y=[1 0 0]*(A0*hat_x+B0*delta_u); 
%     
% else
%     count=mod(t_now,0.05);
%     if(count==0)%在采样的时刻
%         predict_y=y_real;
%         hat_x=A_bar*hat_x_last +B_bar*delta_u_last+ C_bar*predict_y;
%         %hat_x(1,1)=y_real;
%         [u, delta_u, mu, mu_p, mu_pp]  = AIC3(t_now, 1, y_real,hat_x(1,1),y2_derivative_sampling,hat_x(2,1), y3_real_slow, hat_x(3,1), mu_last, mu_p_last, mu_pp_last, u_last);
% 
%         %predict_y=[1 0 0]*(A0*hat_x+B0*delta_u);
%         
%     else%在两个采样时刻之间
%         predict_y=[1 0 0]*(A0*hat_x_last+B0*delta_u_last);
%         hat_x=A_bar*hat_x_last + B_bar*delta_u_last+C_bar*predict_y_last;
%         [u, delta_u, mu, mu_p, mu_pp]  = AIC3(t_now, 1, y_real,hat_x(1,1),y2_derivative_sampling,hat_x(2,1), y3_real_slow, hat_x(3,1), mu_last, mu_p_last, mu_pp_last, u_last);
%         %predict_y=[1 0 0]*(A0*hat_x+B0*delta_u);
%         
%     end
% end
% end

== matlab function ur5_simulink_ros2_pbvs_aic/MATLAB Function4 ==
  data: y output
function y = fcn()
    y =zeros(1,4);
    y(1) = 0.0;
    y(2) = 0.7071;
    y(3) = -0.7071;
    y(4) = 0.0;
end

== matlab function ur5_simulink_ros2_pbvs_aic/Subsystem/MATLAB Function ==
  data: u input; x output; y output; z output
function [x,y,z]= fcn(u)
x = u(1);
y = u(2);
z = u(3);

== matlab function ur5_simulink_ros2_pbvs_aic/ROS2 Time Generator/MATLAB Function ==
  data: current_time input; last_time input; time_x output; init_time output
function [time_x,init_time] = fcn(current_time, last_time)
init_time = last_time;
time_x = current_time-last_time;

== matlab function ur5_simulink_ros2_pbvs_aic/Subsystem5/attitude_pi_ctrl/Subsystem/MATLAB Function ==
  data: R_current input; u output; Ts input
function u  = attitudePIDControl(R_current, Ts)
    % 计算姿态误差矩阵
    Kp=0.5;
    persistent R_target isFirstCall

    % 在第一次调用时初始化
    if isempty(isFirstCall)
        isFirstCall = false;
        R_target = R_current;  % 将当前姿态设置为目标姿态
    end

    sym_ref = [0,-R_target(4),R_target(3);R_target(4),0,-R_target(2);-R_target(3),R_target(2),0];
    current_error_quat =R_current(1)*R_target(2:4)'-R_target(1)*R_current(2:4)'-sym_ref*R_current(2:4)';
    u=(Kp*current_error_quat); 
end

== matlab function ur5_simulink_ros2_pbvs_aic/Error generator ==
  data: refer_quat input; ee_current input; obj_position input; current_error output
function current_error  = fcn(refer_quat, ee_current, obj_position)
    position_error = zeros(3,1);
    current_quat = ee_current(4:7);
    ref_quat = refer_quat;
    sym_ref = [0,-ref_quat(4),ref_quat(3);ref_quat(4),0,-ref_quat(2);-ref_quat(3),ref_quat(2),0];
    current_error_quat =current_quat(1)*ref_quat(2:4)-ref_quat(1)*current_quat(2:4)-sym_ref*current_quat(2:4);
    position_error(1) = -0.1-1*(ee_current(1)-obj_position(1));
    position_error(2) = -0.02-1*(ee_current(2)-obj_position(2));
    position_error(3) = 0.3-1*(ee_current(3)-obj_position(3));
    current_error = [1*position_error; 0.0*current_error_quat];% x y z

end

== matlab function ur5_simulink_ros2_pbvs_aic/PID Controller ==
  data: jacobian_matrix input; y output; current_error input
function y = fcn(jacobian_matrix, current_error)
    y = jacobian_matrix\current_error;
end

== matlab function ur5_simulink_ros2_pbvs_aic/MATLAB Function3 ==
  data: camera_rot input; obj_pos input; y output
function y = fcn(camera_rot, obj_pos)
    temp_pos = [obj_pos(1);obj_pos(2);obj_pos(3);1];
    new_pos = camera_rot*temp_pos;
    y = new_pos(1:3);
end

== matlab function ur5_simulink_ros2_pbvs_aic/joint vel to ros3/to ros2 ==
  data: u input; flag input; y output; joint1 input; joint2 input; joint3 input; joint4 input; joint5 input; joint6 input
function y  = fcn(u,flag, joint1, joint2, joint3, joint4, joint5, joint6)
    y = zeros(128,1);
    if(flag==0)
        y(1) = u(1);
        y(2) = u(2);
        y(3) = u(3);
        y(4) = u(4);
        y(5) = u(5);
        y(6) = u(6);
    else
        y(1) = joint1;
        y(2) = joint2;
        y(3) = joint3;
        y(4) = joint4;
        y(5) = joint5;
        y(6) = joint6;
    end
end

== matlab function ur5_simulink_ros2_pbvs_aic/APO+AIC/Subsystem1/APO+AIC/MATLAB Function ==
  data: count output; hat_x_last input; predict_y_last input; y_real input; y2_derivative_sampling input; u_last input; delta_u_last input; hat_x output; t_now input; A_bar input; B_bar input; C_bar input; predict_y output; A0 input; B0 input; mu_last input; mu_p_last input; u output; delta_u output; mu output; mu_p output
function [count,hat_x,predict_y, u, delta_u, mu, mu_p] = fcn(hat_x_last, predict_y_last, y_real,y2_derivative_sampling, u_last,delta_u_last,t_now,A_bar,B_bar,C_bar,A0,B0,mu_last, mu_p_last)
if(t_now==0)
    count=0;
    hat_x = zeros(2,1);
    predict_y = y_real;
    hat_x(1,1)=y_real;
    [u, delta_u, mu, mu_p]  = AIC2(t_now, 1, y_real,hat_x(1,1),y2_derivative_sampling,hat_x(2,1), mu_last, mu_p_last, u_last);
else
    count=mod(t_now,0.05);
    if(count==0)%在采样的时刻
        predict_y=y_real;
        hat_x=A_bar*hat_x_last +B_bar*delta_u_last/0.01+ C_bar*predict_y;
        [u, delta_u, mu, mu_p]  = AIC2(t_now, 1, y_real,hat_x(1,1),y2_derivative_sampling,hat_x(2,1), mu_last, mu_p_last, u_last);
    else%在两个采样时刻之间
        predict_y=[1 0]*(A0*hat_x_last+B0*delta_u_last);
        hat_x=A_bar*hat_x_last + B_bar*delta_u_last/0.01+C_bar*predict_y_last;
        [u, delta_u, mu, mu_p]  = AIC2(t_now, 1, y_real,hat_x(1,1),y2_derivative_sampling,hat_x(2,1), mu_last, mu_p_last, u_last);
    end
end
end








% function [count,hat_x,predict_y, u, delta_u, mu, mu_p, mu_pp] = fcn(hat_x_last, predict_y_last, y_real,y2_derivative_sampling,y3_real_slow, u_last,delta_u_last,t_now,A_bar,B_bar,C_bar,A0,B0,mu_last, mu_p_last, mu_pp_last)
% if(t_now==0)
%     count=0;
%     hat_x = zeros(3,1);
%     predict_y = y_real;
%     hat_x(1,1)=y_real;
%     u_now=0;
%     hat_x = A_bar*hat_x + B_bar*u_now+ C_bar*predict_y;
%     [u, delta_u, mu, mu_p, mu_pp]  = AIC3(t_now, 1, y_real,hat_x(1,1),y2_derivative_sampling,hat_x(2,1), y3_real_slow, hat_x(3,1), mu_last, mu_p_last, mu_pp_last, u_last);
%     %predict_y=[1 0 0]*(A0*hat_x+B0*delta_u); 
%     
% else
%     count=mod(t_now,0.05);
%     if(count==0)%在采样的时刻
%         predict_y=y_real;
%         hat_x=A_bar*hat_x_last +B_bar*delta_u_last+ C_bar*predict_y;
%         %hat_x(1,1)=y_real;
%         [u, delta_u, mu, mu_p, mu_pp]  = AIC3(t_now, 1, y_real,hat_x(1,1),y2_derivative_sampling,hat_x(2,1), y3_real_slow, hat_x(3,1), mu_last, mu_p_last, mu_pp_last, u_last);
% 
%         %predict_y=[1 0 0]*(A0*hat_x+B0*delta_u);
%         
%     else%在两个采样时刻之间
%         predict_y=[1 0 0]*(A0*hat_x_last+B0*delta_u_last);
%         hat_x=A_bar*hat_x_last + B_bar*delta_u_last+C_bar*predict_y_last;
%         [u, delta_u, mu, mu_p, mu_pp]  = AIC3(t_now, 1, y_real,hat_x(1,1),y2_derivative_sampling,hat_x(2,1), y3_real_slow, hat_x(3,1), mu_last, mu_p_last, mu_pp_last, u_last);
%         %predict_y=[1 0 0]*(A0*hat_x+B0*delta_u);
%         
%     end
% end
% end
